simulink model "ej1b"  (R2020b)
settings: Solver=VariableStepAuto  StartTime=0.0  StopTime=10.0  RelTol=1e-3
settings Model: Creator=Kike  LastModifiedBy=zunt7

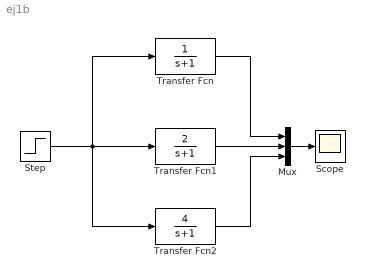
== system ej1b ==
  Mux : Mux  Inputs=3
  Scope : Scope
  Step : Step  Time=0  SampleTime=0
  Transfer Fcn : TransferFcn  Denominator=[1 1]
  Transfer Fcn1 : TransferFcn  Numerator=[2]  Denominator=[1 1]
  Transfer Fcn2 : TransferFcn  Numerator=[4]  Denominator=[1 1]
  wires:
  Step/1 -> Transfer Fcn2/1, Transfer Fcn1/1, Transfer Fcn/1
  Transfer Fcn1/1 -> Mux/2
  Mux/1 -> Scope/1
  Transfer Fcn/1 -> Mux/1
  Transfer Fcn2/1 -> Mux/3
